simulink model "adc_power_inl"  (R2013a)
settings: Solver=VariableStepDiscrete  StartTime=0.0  StopTime=1.0  RelTol=1e-3
undefined symbols (not defined in the file or in its folder): get, One, sided
libraries: dspsrcs4 x1, dspsnks4 x1
settings Model: Creator=bbhattac  LastModifiedBy=bbhattac
settings OptimizationCC: ExpressionDepthLimit=2147483647
settings DebuggingCC: ParameterPrecisionLossMsg=none  FcnCallInpInsideContextMsg=UseLocalSettings
settings GRTTargetCC: CombineOutputUpdateFcns=off  GRTInterface=on

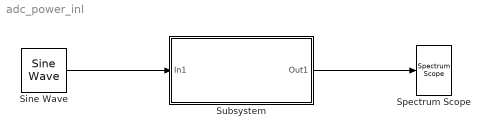
== system adc_power_inl ==
  Sine Wave : dspsrcs4/Sine Wave  Amplitude=1  Frequency=10000  Phase=0  SampleMode=Discrete  OutComplex=Real  CompMethod=Trigonometric fcn  TableSize=Speed  SampleTime=1/200000  SamplesPerFrame=1  ResetState=Restart at time zero  dataType=double  wordLen=16  udDataType=sfix(16)  fracBitsMode=Best precision  numFracBits=15  OutDataTypeStr=double  LastOutDataTypeStr=double
  Spectrum Scope : dspsnks4/Spectrum Scope  SystemSampleTime=-1  ScopeProperties=on  Domain=Frequency  HorizSpan=1  UseBuffer=on  BufferSize=1024  Overlap=0  inpFftLenInherit=off  FFTlength=128  numAvg=2  DisplayProperties=off  AxisGrid=on  Memory=off  FrameNumber=on  AxisLegend=off  AxisZoom=off  OpenScopeAtSimStart=on  OpenScopeImmediately=off  FigPos=get(0,'defaultfigureposition')  AxisProperties=off  XUnits=Hertz  XRange=One-sided ([0...Fs/2])  XDisplay=0  InheritXIncr=on  XIncr=1.0  XLabel=Samples  XLimit=User-defined  YUnits=dBW/Hertz  XMax=100000  XMin=0  YLabel=Magnitude-squared, dB  LineProperties=off  wintypeSpecScope=Hann  RsSpecScope=50  betaSpecScope=5  winsampSpecScope=Periodic  XAxisParamsVer=6.9
      settings: YMin=-208.0331  YMax=-16.4509
  Subsystem : Subsystem  mask(Power Series Nonlinearity){nonlingain=1e-05, mu=1e-07}
      mask prompts: nonlingain "Nonlinear factor"; mu "Asymmetry factor"
      mask help: Models the integral nonlinearity of an ADC using 1st order power series.
      mask Help:
      | This block models the integral nonlinearity of an A/D converter using a 1st order power series.
      | Typical values for a high resolution (16 bits or higher) ADC are:
      |   Nonlinear factor = 1.0e-05;
      |   Asymmetry factor = 1.0e-05;
      | 
      | Ref: "Analog-to-Digital Conversion and Harmonic Noises Due to the Integral Nonlinearity," Kiseon Kim, IEEE Trans. Inst. and Meas. Vol. 43, No. 2, pp. 151-156.
      mask Display: disp('Power Series\n Nonlinearity');
  wires:
  Sine Wave/1 -> Subsystem/1(In1)
  Subsystem/1(Out1) -> Spectrum Scope/1

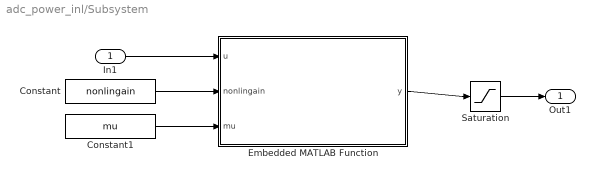
== system adc_power_inl/Subsystem ==
  In1 : Inport
  Constant : Constant  Value=nonlingain  VectorParams1D=off
  Constant1 : Constant  Value=mu  VectorParams1D=off
  Embedded MATLAB Function : MATLAB Function  TreatAsAtomicUnit=on
  Saturation : Saturate  UpperLimit=1.0  LowerLimit=-1.0
  Out1 : Outport
  wires:
  Embedded MATLAB Function/1(y) -> Saturation/1
  In1/1 -> Embedded MATLAB Function/1(u)
  Saturation/1 -> Out1/1
  Constant/1 -> Embedded MATLAB Function/2(nonlingain)
  Constant1/1 -> Embedded MATLAB Function/3(mu)

== matlab function adc_power_inl/Subsystem/Embedded MATLAB Function ==
  data: u input; y output; nonlingain input; mu input
function y = ADC_INL(u,nonlingain,mu)
%#eml

if u==0
    y = 0;
elseif u>0
    y = u^(1-nonlingain) + mu*(u^2);
else
    y = -(-u)^(1-nonlingain) + mu*(u^2);
end
